simulink model "Udan_SOC"  (R2017b)
settings: Solver=FixedStepAuto  StartTime=0.0  StopTime=1000  FixedStep=0.1  RelTol=1e-3
values from neighbouring files (symbols this model uses):
  DenominatorOfIntegratorFactor = 100.0    [SOC_Stateflow.sldd]
  SOC_CalcSohLKT = 1.0    [SOC_Stateflow.sldd]
  SOC_CalcSOHTempLimit = 70.0    [SOC_Stateflow.sldd]
  SOC_CapPerCycle = 100.0    [SOC_Stateflow.sldd]
  SOC_CapTemp_HLimit = 200.0    [SOC_Stateflow.sldd]
  SOC_CapTemp_LLimit = 0.0    [SOC_Stateflow.sldd]
  Soc_ConfigInfo = 0    [SOC_Stateflow.sldd]
  SOC_DchgEndCalib = 0.0    [SOC_Stateflow.sldd]
  SOC_DiffVoltMin = 10.0    [SOC_Stateflow.sldd]
  SOC_DSOCJumpMax = 500.0    [SOC_Stateflow.sldd]
  SOC_EfficientHighLimit = 250.0    [SOC_Stateflow.sldd]
  SOC_EfficientLowLimit = 40.0    [SOC_Stateflow.sldd]
  SOC_EmptyAus = 0.0    [SOC_Stateflow.sldd]
  SOC_EnableOcv = 1.0    [SOC_Stateflow.sldd]
  SOC_END_CALIB_STATE : value not decoded    [SOC_Stateflow.sldd]
  SOC_HighRealSoc = 95.0    [SOC_Stateflow.sldd]
  SOC_LKTSohCycles = 0.0 1.0 10.0 20.0 30.0 40.0 50.0 60.0 70.0 80.0 90.0 100.0 110.0 120.0 130.0 140.0 150.0 160.0 170.0 180.0 190.0 200.0 210.0 220.0 230.0 240.0 250.0 260.0 270.0 280.0 290.0 300.0 310.0 320.0 330.0 340.0 350.0 360.0 370.0 380.0 390.0 400.0 410.0 420.0 430.0 440.0 450.0 460.0 470.0 480.0 490.0 500.0 510.0 520.0 530.0 540.0 550.0 560.0 570.0 580.0 590.0 600.0 610.0 620.0 630.0 640.0 650.0 660.0 670.0    [SOC_Stateflow.sldd]
  SOC_LKTSohTable = 1000.0 991.0 989.0 992.0 993.0 995.0 994.0 993.0 1000.0 997.0 1002.0 1000.0 992.0 1000.0 989.0 992.0 989.0 994.0 989.0 993.0 994.0 994.0 994.0 993.0 991.0 991.0 992.0 993.0 991.0 985.0 985.0 985.0 979.0 975.0 978.0 984.0 982.0 974.0 975.0 972.0 972.0 975.0 977.0 977.0 974.0 971.0 973.0 971.0 966.0 968.0 965.0 959.0 957.0 956.0 957.0 954.0 955.0 951.0 954.0 951.0 942.0 942.0 940.0 942.0 947.0 949.0    [SOC_Stateflow.sldd]
  SOC_LowRealSoc = 5.0    [SOC_Stateflow.sldd]
  SOC_NominalCap_AmS = 576000000.0    [SOC_Stateflow.sldd]
  SOC_NominalVol = 4000.0    [SOC_Stateflow.sldd]
  SOC_OCVTemp_HLimit = 106.0    [SOC_Stateflow.sldd]
  SOC_OCVTemp_LLimit = 29.0    [SOC_Stateflow.sldd]
  SOC_ShortCalibDSoc = 1.0    [SOC_Stateflow.sldd]
  SOC_SOCResolution = 10000.0    [SOC_Stateflow.sldd]
  SOC_SohCalcCapPercent = 8.0    [SOC_Stateflow.sldd]
  SOC_SohCalcHighLimit = 60.0    [SOC_Stateflow.sldd]
  SOC_SohCalcLowLimit = 10.0    [SOC_Stateflow.sldd]
  SOC_SohCalcMidLimit = 30.0    [SOC_Stateflow.sldd]
  SOC_SOHResolution = 1000.0    [SOC_Stateflow.sldd]
  SOC_State = <binary blob, 1163 chars, not shown>    [SOC_Stateflow.sldd]
  SOC_TempCap_CapBuffer : value not decoded    [SOC_Stateflow.sldd]
  SOC_TempCap_TempBuffer : value not decoded    [SOC_Stateflow.sldd]
  SocOcvCalib_ConfigInfo = 0.0    [SOC_Stateflow.sldd]
  SocOcvCalib_SocBuffer1 : value not decoded    [SOC_Stateflow.sldd]
  SocOcvCalib_TempBuffer : value not decoded    [SOC_Stateflow.sldd]
  SocOcvCalib_VoltageBuffer1 = 3300.0 3303.0 3305.0 3307.0 3310.0 3311.0 3313.0 3314.0 3316.0 3317.0 3319.0 3320.0 3322.0 3323.0 3325.0 3322.0 3323.0 3325.0 3310.0 3313.0 3315.0 3317.0 3320.0 3321.0 3323.0 3324.0 3326.0 3327.0 3329.0 3330.0 3332.0 3333.0 3335.0 3332.0 3333.0 3335.0 3320.0 3323.0 3325.0 3327.0 3330.0 3331.0 3333.0 3334.0 3336.0 3337.0 3339.0 3340.0 3342.0 3343.0 3345.0 3342.0 3343.0 3345.0 3330.0 3333.0 3335.0 3    [SOC_Stateflow.sldd]
  SOHCalibCycle = 10.0    [SOC_Stateflow.sldd]
undefined symbols (not defined in the file or in its folder): DatetimeM_GetReturnType, ParameterM_EeepParaIndexType, Soc_CumuLativeTypeType, SOC_EgthTempChgValue, Soc_EnergyBuffer, SOC_FithTempChgValue, SOC_FstSlowTempChgValue, SOC_FstTempChgValue, SOC_FthTempChgValue, SOC_MaxCap_AmS, SOC_SethTempChgValue, SOC_SixTempChgValue, SOC_SndSlowTempChgValue, SOC_SndTempChgValue, SOC_TrdSlowTempChgValue, SOC_TrdTempChgValue, SocDiagCalib_NoCalibReasonType
libraries: simulink x138, hdlsllib x24, dspindex x4
(part 3 of 10)

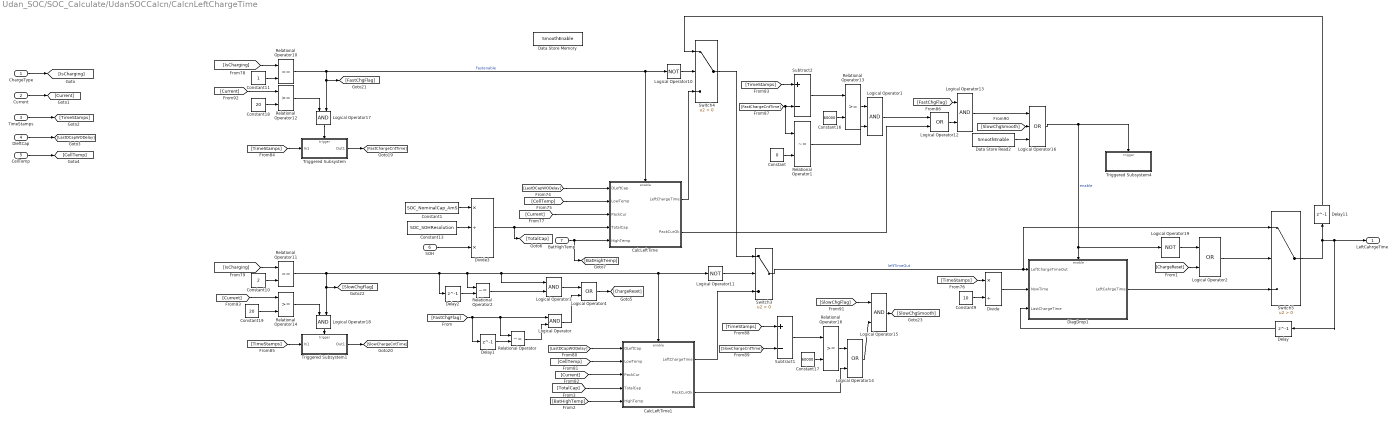
== system Udan_SOC/SOC_Calculate/UdanSOCCalcn/CalcnLeftChargeTime ==
  ChargeType : Inport
  Current : Inport  Port=2
  TimeStamps : Inport  Port=3
  DleftCap : Inport  Port=4
  CellTemp : Inport  Port=5
  SOH : Inport  Port=6
  BatHighTemp : Inport  Port=7
  CalcLeftTime : Subsystem
  CalcLeftTime1 : Subsystem
  Constant : Constant  Value=0  OutDataTypeStr=uint8
  Constant1 : Constant  Value=SOC_NominalCap_AmS
  Constant10 : Constant  Value=2  OutDataTypeStr=uint8
  Constant11 : Constant  OutDataTypeStr=uint8
  Constant13 : Constant  Value=SOC_SOHResolution  OutDataTypeStr=uint16
  Constant16 : Constant  Value=60000  OutDataTypeStr=uint16
  Constant17 : Constant  Value=60000  OutDataTypeStr=uint16
  Constant18 : Constant  Value=20  OutDataTypeStr=uint8
  Constant19 : Constant  Value=20  OutDataTypeStr=uint8
  Constant9 : Constant  Value=10  OutDataTypeStr=uint8
  Data Store Memory : DataStoreMemory  DataStoreName=SmoothEnable  ReadBeforeWriteMsg=warning  WriteAfterWriteMsg=warning  WriteAfterReadMsg=warning  ShowAdditionalParam=off  OutDataTypeStr=boolean
  Data Store Read2 : DataStoreRead  DataStoreName=SmoothEnable
  Delay{,1..2,11} (4 alike) : Delay  DelayLength=1  InitialCondition=0
  DiagDrop1 : Subsystem  mask(DiagDrop(UDAN Lib)){}
      mask help: This block is used to void the slump
  Divide : Product  Inputs=*/  OutDataTypeStr=uint32
  Divide3 : Product  Inputs=*/*  OutDataTypeStr=uint32
  Logical Operator{,1,3,13,15,17..18} (7 alike) : Logic  AllPortsSameDT=off  OutDataTypeStr=boolean
  Logical Operator10 : Logic  Operator=NOT  AllPortsSameDT=off  OutDataTypeStr=boolean
  Logical Operator11 : Logic  Operator=NOT  AllPortsSameDT=off  OutDataTypeStr=boolean
  Logical Operator{2,4,12,14} (4 alike) : Logic  Operator=OR  AllPortsSameDT=off  OutDataTypeStr=boolean
  Logical Operator16 : Logic  Operator=OR  Inputs=3  AllPortsSameDT=off  OutDataTypeStr=boolean
  Logical Operator19 : Logic  Operator=NOT  AllPortsSameDT=off  OutDataTypeStr=boolean
  Relational Operator : RelationalOperator  Operator=~=  OutDataTypeStr=boolean  RndMeth=Simplest
  Relational Operator1 : RelationalOperator  Operator=~=  OutDataTypeStr=boolean  RndMeth=Simplest
  Relational Operator10 : RelationalOperator  Operator===  OutDataTypeStr=boolean  RndMeth=Simplest
  Relational Operator11 : RelationalOperator  Operator===  OutDataTypeStr=boolean  RndMeth=Simplest
  Relational Operator{12..14,16} (4 alike) : RelationalOperator  OutDataTypeStr=boolean  RndMeth=Simplest
  Relational Operator2 : RelationalOperator  Operator=~=  OutDataTypeStr=boolean  RndMeth=Simplest
  Subtract1 : Sum  Inputs=+-  AccumDataTypeStr=uint32  OutDataTypeStr=uint32
  Subtract2 : Sum  Inputs=+-  AccumDataTypeStr=uint32  OutDataTypeStr=uint32
  Switch3 : Switch  Criteria=u2 > Threshold
  Switch4 : Switch  Criteria=u2 > Threshold
  Switch5 : Switch  Criteria=u2 > Threshold
  Triggered Subsystem : Subsystem  TreatAsAtomicUnit=on
  Triggered Subsystem1 : Subsystem  TreatAsAtomicUnit=on
  Triggered Subsystem4 : Subsystem  TreatAsAtomicUnit=on
  LeftCahrgeTime : Outport
  wires:
  Logical Operator2/1 -> Switch5/2
  Logical Operator/1 -> Logical Operator4/2
  Delay1/1 -> Relational Operator/2
  Relational Operator/1 -> Logical Operator/2
  [FastChgFlag] -> Logical Operator/1, Relational Operator/1, Delay1/1
  Delay/1 -> DiagDrop1/3(LastChargeTime)
  Delay11/1 -> Switch4/1
  Switch4/1 -> Switch3/1
  CalcLeftTime/2(PackCurOk) -> Logical Operator12/2
  [Current] -> CalcLeftTime/3(PackCur)
  Relational Operator10/1 -> Logical Operator17/2, [FastChgFlag], Logical Operator10/1, CalcLeftTime/Enable  "Fastenable"
  Constant9/1 -> Divide/2
  [IsCharging] -> Relational Operator10/1
  Constant11/1 -> Relational Operator10/2
  Constant10/1 -> Relational Operator11/2
  Subtract2/1 -> Relational Operator13/1
  Switch5/1 -> Delay11/1, LeftCahrgeTime/1, Delay/1
  [FastChargeCntTime] -> Relational Operator1/1, Subtract2/2
  Relational Operator13/1 -> Logical Operator1/1
  Logical Operator10/1 -> Switch4/2
  [IsCharging] -> Relational Operator11/1
  [Current] -> CalcLeftTime1/3(PackCur)
  [LastDCapWODelay] -> CalcLeftTime1/1(DLeftCap)
  [LastDCapWODelay] -> CalcLeftTime/1(DLeftCap)
  [TimeStamps] -> Triggered Subsystem1/1(In1)
  Triggered Subsystem1/1(Out1) -> [SlowChargeCntTime]
  Triggered Subsystem/1(Out1) -> [FastChargeCntTime]
  [TimeStamps] -> Subtract2/1
  [CellTemp] -> CalcLeftTime1/2(LowTemp)
  Constant16/1 -> Relational Operator13/2
  [CellTemp] -> CalcLeftTime/2(LowTemp)
  Logical Operator15/1 -> [SlowChgSmooth]
  DiagDrop1/1(LeftCahrgeTime) -> Switch5/3
  Switch3/1 -> Switch5/1, DiagDrop1/1(LeftChargeTimeOut)  "leftTimeOut"
  Logical Operator18/1 -> Triggered Subsystem1/Trigger
  Logical Operator13/1 -> Logical Operator16/1
  Logical Operator17/1 -> Triggered Subsystem/Trigger
  [TimeStamps] -> Divide/1
  Relational Operator12/1 -> Logical Operator17/1
  [Current] -> Relational Operator14/1
  [Current] -> Relational Operator12/1
  Constant18/1 -> Relational Operator12/2
  [SlowChgSmooth] -> Logical Operator16/2
  Relational Operator14/1 -> Logical Operator18/1
  Logical Operator19/1 -> Logical Operator2/1
  Logical Operator16/1 -> Triggered Subsystem4/Trigger, Logical Operator19/1, DiagDrop1/Enable  "enable"
  Constant19/1 -> Relational Operator14/2
  [TimeStamps] -> Triggered Subsystem/1(In1)
  Divide/1 -> DiagDrop1/2(NowTime)
  [SlowChargeCntTime] -> Subtract1/2
  CalcLeftTime1/2(PackCurOk) -> Logical Operator14/2
  CalcLeftTime/1(LeftChargeTime) -> Switch4/3
  Logical Operator14/1 -> Logical Operator15/2
  [TimeStamps] -> Subtract1/1
  Relational Operator16/1 -> Logical Operator14/1
  [SlowChgFlag] -> Logical Operator15/1
  Subtract1/1 -> Relational Operator16/1
  Constant17/1 -> Relational Operator16/2
  CalcLeftTime1/1(LeftChargeTime) -> Switch3/3
  Logical Operator12/1 -> Logical Operator13/2
  Logical Operator11/1 -> Switch3/2
  [FastChgFlag] -> Logical Operator13/1
  ChargeType/1 -> [IsCharging]
  Current/1 -> [Current]
  TimeStamps/1 -> [TimeStamps]
  DleftCap/1 -> [LastDCapWODelay]
  CellTemp/1 -> [CellTemp]
  Constant/1 -> Relational Operator1/2
  Relational Operator1/1 -> Logical Operator1/2
  Logical Operator1/1 -> Logical Operator12/1
  Data Store Read2/1 -> Logical Operator16/3
  Relational Operator11/1 -> Delay2/1, Relational Operator2/1, Logical Operator3/1, CalcLeftTime1/Enable, Logical Operator11/1, [SlowChgFlag], Logical Operator18/2
  Delay2/1 -> Relational Operator2/2
  Relational Operator2/1 -> Logical Operator3/2
  Logical Operator3/1 -> Logical Operator4/1
  Logical Operator4/1 -> [ChargeReset]
  [ChargeReset] -> Logical Operator2/2
  SOH/1 -> Divide3/3
  [TotalCap] -> CalcLeftTime1/4(TotalCap)
  Constant13/1 -> Divide3/2
  Constant1/1 -> Divide3/1
  Divide3/1 -> [TotalCap], CalcLeftTime/4(TotalCap)
  BatHighTemp/1 -> [BatHighTemp], CalcLeftTime/5(HighTemp)
  [BatHighTemp] -> CalcLeftTime1/5(HighTemp)

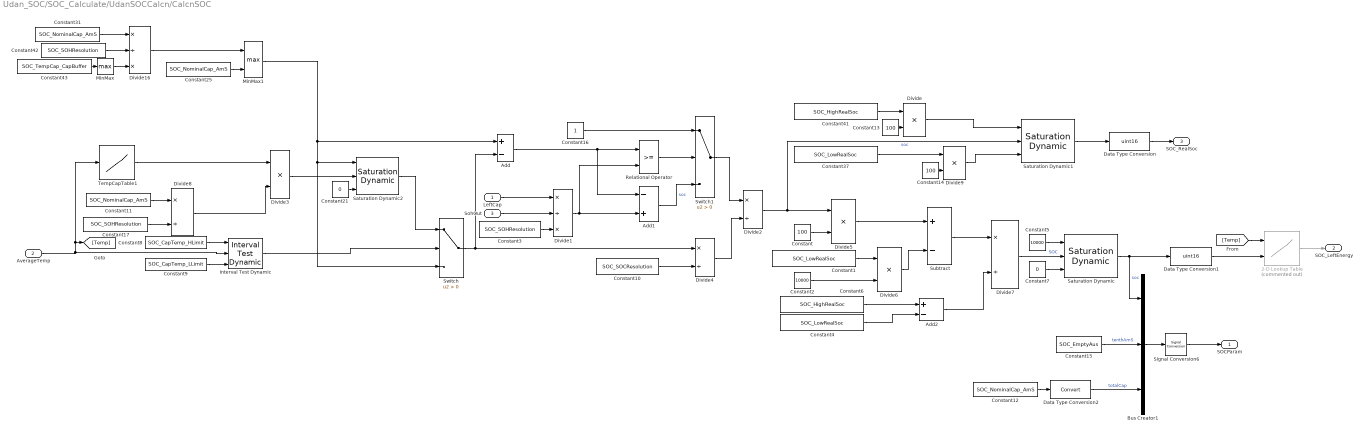
== system Udan_SOC/SOC_Calculate/UdanSOCCalcn/CalcnSOC ==
  LeftCap : Inport
  AverageTemp : Inport  Port=2
  SohOut : Inport  Port=3
  2-D Lookup Table : Lookup_n-D  Commented=on  BreakpointsForDimension1=SocOcvCalib_TempBuffer  BreakpointsForDimension2=SocOcvCalib_SocBuffer1  Table=Soc_EnergyBuffer  ExtrapMethod=Clip  InternalRulePriority=Speed  OutDataTypeStr=uint16  RndMeth=Simplest
  Add : Sum  Inputs=+-
  Add1 : Sum  Inputs=-+  AccumDataTypeStr=uint32  OutDataTypeStr=uint32
  Add2 : Sum  Inputs=+-  AccumDataTypeStr=uint8  OutDataTypeStr=uint8
  Bus Creator1 : BusCreator  Inputs=3  OutDataTypeStr=Bus: SOX_SocType
      settings: InheritFromInputs=off
  Constant : Constant  Value=100  OutDataTypeStr=uint8
  Constant1 : Constant  Value=SOC_LowRealSoc
  Constant10 : Constant  Value=SOC_SOCResolution  OutDataTypeStr=uint16
  Constant{11..12,25,31} (4 alike) : Constant  Value=SOC_NominalCap_AmS
  Constant13 : Constant  Value=100  OutDataTypeStr=uint8
  Constant14 : Constant  Value=100  OutDataTypeStr=uint8
  Constant15 : Constant  Value=SOC_EmptyAus
  Constant16 : Constant  OutDataTypeStr=uint32
  Constant17 : Constant  Value=SOC_SOHResolution  OutDataTypeStr=uint16
  Constant2 : Constant  Value=10000  OutDataTypeStr=uint16
  Constant21 : Constant  Value=0  OutDataTypeStr=uint8
  Constant3 : Constant  Value=SOC_SOHResolution  OutDataTypeStr=uint16
  Constant37 : Constant  Value=SOC_LowRealSoc
  Constant4 : Constant  Value=SOC_LowRealSoc
  Constant41 : Constant  Value=SOC_HighRealSoc
  Constant42 : Constant  Value=SOC_SOHResolution  OutDataTypeStr=uint16
  Constant43 : Constant  Value=SOC_TempCap_CapBuffer
  Constant5 : Constant  Value=10000  OutDataTypeStr=uint16
  Constant6 : Constant  Value=SOC_HighRealSoc
  Constant7 : Constant  Value=0  OutDataTypeStr=uint16
  Constant8 : Constant  Value=SOC_CapTemp_HLimit  OutDataTypeStr=uint8
  Constant9 : Constant  Value=SOC_CapTemp_LLimit  OutDataTypeStr=uint8
  Data Type Conversion : DataTypeConversion  OutDataTypeStr=uint16
  Data Type Conversion1 : DataTypeConversion  OutDataTypeStr=uint16
  Data Type Conversion2 : DataTypeConversion
  Divide : Product  Inputs=**
  Divide1 : Product  Inputs=*/*  OutDataTypeStr=uint32
  Divide16 : Product  Inputs=*/*  OutDataTypeStr=uint32
  Divide2 : Product  Inputs=*/  OutDataTypeStr=int32
  Divide3 : Product  Inputs=**  OutDataTypeStr=uint32
  Divide4 : Product  Inputs=*/  OutDataTypeStr=int32
  Divide5 : Product  Inputs=**  OutDataTypeStr=uint32
  Divide6 : Product  Inputs=**  OutDataTypeStr=uint32
  Divide7 : Product  Inputs=*/  OutDataTypeStr=int32
  Divide8 : Product  Inputs=*/  OutDataTypeStr=uint32
  Divide9 : Product  Inputs=**
  Interval Test Dynamic : simulink/Logic and Bit Operations/Interval Test Dynamic  IntervalClosedRight=off  IntervalClosedLeft=off  OutDataTypeStr=boolean
      settings: SourceProductName=Simulink  SourceProductBaseCode=SL
  MinMax : MinMax  Function=max
  MinMax1 : MinMax  Function=max  Inputs=2
  Relational Operator : RelationalOperator  OutDataTypeStr=boolean  RndMeth=Simplest
  Saturation Dynamic : simulink/Discontinuities/Saturation Dynamic  OutMin=[]  OutMax=[]  OutDataTypeStr=uint32  OutputDataTypeScalingMode=uint32  OutDataType=fixdt(1, 16)  OutScaling=2^-10  DoSatur=on
  Saturation Dynamic1 : simulink/Discontinuities/Saturation Dynamic  OutMin=[]  OutMax=[]  OutDataTypeStr=uint32  OutputDataTypeScalingMode=uint32  OutDataType=fixdt(1, 16)  OutScaling=2^-10  DoSatur=on
  Saturation Dynamic2 : simulink/Discontinuities/Saturation Dynamic  OutMin=[]  OutMax=[]  OutDataTypeStr=Inherit: Same as second input  OutDataType=fixdt(1, 16)  OutScaling=2^-10  DoSatur=off
  Signal Conversion6 : SignalConversion  ConversionOutput=Nonvirtual bus  OverrideOpt=off
  Subtract : Sum  Inputs=+-  AccumDataTypeStr=int32  OutDataTypeStr=int32
  Switch : Switch  Criteria=u2 > Threshold
  Switch1 : Switch  Criteria=u2 > Threshold  OutDataTypeStr=uint32
  TempCapTable1 : Lookup_n-D  NumberOfTableDimensions=1  BreakpointsForDimension1=SOC_TempCap_TempBuffer  Table=SOC_TempCap_CapBuffer  ExtrapMethod=Clip  InternalRulePriority=Speed  OutDataTypeStr=uint16  RndMeth=Simplest  InputSameDT=on
  SOCParam : Outport
  SOC_LeftEnergy : Outport  Port=2
  SOC_RealSoc : Outport  Port=3
  wires:
  Constant15/1 -> Bus Creator1/2  "tenthAmS"
  LeftCap/1 -> Divide1/1
  Constant10/1 -> Divide4/2
  TempCapTable1/1 -> Divide3/1
  Constant3/1 -> Divide1/3
  Divide7/1 -> Saturation Dynamic/2  "SOC"
  Constant7/1 -> Saturation Dynamic/3
  Constant5/1 -> Saturation Dynamic/1
  SohOut/1 -> Divide1/2
  Saturation Dynamic/1 -> Data Type Conversion1/1, Bus Creator1/1  "soc"
  Divide4/1 -> Divide2/2
  Signal Conversion6/1 -> SOCParam/1
  Bus Creator1/1 -> Signal Conversion6/1
  Switch/1 -> Add/2, Divide4/1
  Divide8/1 -> Divide3/2
  AverageTemp/1 -> [Temp], TempCapTable1/1, Interval Test Dynamic/2
  Constant9/1 -> Interval Test Dynamic/3
  Constant8/1 -> Interval Test Dynamic/1
  Interval Test Dynamic/1 -> Switch/2
  Saturation Dynamic2/1 -> Switch/1
  MinMax1/1 -> Add/1, Saturation Dynamic2/1, Switch/3
  Divide1/1 -> Relational Operator/2, Add1/2
  Add/1 -> Add1/1, Relational Operator/1
  Constant17/1 -> Divide8/2
  Divide2/1 -> Divide5/1, Saturation Dynamic1/2  "soc"
  Data Type Conversion1/1 -> 2-D Lookup Table/2
  [Temp] -> 2-D Lookup Table/1
  2-D Lookup Table/1 -> SOC_LeftEnergy/1
  Data Type Conversion/1 -> SOC_RealSoc/1
  Saturation Dynamic1/1 -> Data Type Conversion/1
  Divide3/1 -> Saturation Dynamic2/2
  Constant21/1 -> Saturation Dynamic2/3
  Constant/1 -> Divide5/2
  Divide5/1 -> Subtract/1
  Constant2/1 -> Divide6/2
  Divide6/1 -> Subtract/2
  Subtract/1 -> Divide7/1
  Add2/1 -> Divide7/2
  Constant13/1 -> Divide/2
  Divide/1 -> Saturation Dynamic1/1
  Constant14/1 -> Divide9/2
  Divide9/1 -> Saturation Dynamic1/3
  Data Type Conversion2/1 -> Bus Creator1/3  "totalCap"
  Constant11/1 -> Divide8/1
  Constant12/1 -> Data Type Conversion2/1
  Constant41/1 -> Divide/1
  Constant37/1 -> Divide9/1
  Constant1/1 -> Divide6/1
  Constant6/1 -> Add2/1
  Constant4/1 -> Add2/2
  Relational Operator/1 -> Switch1/2
  Constant16/1 -> Switch1/1
  Add1/1 -> Switch1/3  "soc"
  Switch1/1 -> Divide2/1
  Constant42/1 -> Divide16/2
  Constant43/1 -> MinMax/1
  MinMax/1 -> Divide16/3
  Divide16/1 -> MinMax1/1
  Constant25/1 -> MinMax1/2
  Constant31/1 -> Divide16/1

== system Udan_SOC/SOC_Calculate/UdanSOCCalcn/CalcnSOC1 ==
  LeftCap : Inport
  Current : Inport  Port=2
  FullCharge : Inport  Port=3
  AverageTemp : Inport  Port=4
  SohOut : Inport  Port=5
  TempCapResolution : Inport  Port=6
  IsCharging : Inport  Port=7
  Abs : Abs
  Add : Sum  Inputs=+-
  Add1 : Sum  Inputs=-+  AccumDataTypeStr=uint32  OutDataTypeStr=uint32
  Bus Creator1 : BusCreator  Inputs=3  OutDataTypeStr=Bus: SOX_SocType
      settings: InheritFromInputs=off
  Constant1 : Constant  Commented=on  Value=10000  OutDataTypeStr=uint16
  Constant10 : Constant  Value=SOC_SOCResolution  OutDataTypeStr=uint16
  Constant{4,6,11,16} (4 alike) : Constant  Value=SOC_NominalCap_AmS
  Constant12 : Constant  Commented=on  Value=9900  OutDataTypeStr=uint16
  Constant13 : Constant  Commented=on  Value=9900  OutDataTypeStr=uint16
  Constant14 : Constant  Value=0  OutDataTypeStr=uint32
  Constant15 : Constant  Value=SOC_EmptyAus
  Constant17 : Constant  Value=SOC_SOHResolution  OutDataTypeStr=uint16
  Constant18 : Constant  Value=SOC_SOHResolution  OutDataTypeStr=uint16
  Constant2 : Constant  Commented=on  Value=2  OutDataTypeStr=int8
  Constant3 : Constant  Value=SOC_SOHResolution  OutDataTypeStr=uint16
  Constant5 : Constant  Value=10000  OutDataTypeStr=uint16
  Constant7 : Constant  Value=0  OutDataTypeStr=uint16
  Constant8 : Constant  Value=SOC_CapTemp_HLimit  OutDataTypeStr=uint8
  Constant9 : Constant  Value=SOC_CapTemp_LLimit  OutDataTypeStr=uint8
  Data Type Conversion : DataTypeConversion
  Delay10 : Delay  Commented=on  DelayLength=1  InitialCondition=0
  Divide1 : Product  Inputs=*/*  OutDataTypeStr=uint32
  Divide2 : Product  Inputs=*/  OutDataTypeStr=int32
  Divide3 : Product  Inputs=**  OutDataTypeStr=uint32
  Divide4 : Product  Inputs=*/  OutDataTypeStr=int32
  Divide8 : Product  Inputs=*/  OutDataTypeStr=uint32
  Interval Test Dynamic : simulink/Logic and Bit Operations/Interval Test Dynamic  IntervalClosedRight=off  IntervalClosedLeft=off  OutDataTypeStr=boolean
      settings: SourceProductName=Simulink  SourceProductBaseCode=SL
  Logical Operator : Logic  Commented=on  Operator=NOT  AllPortsSameDT=off  OutDataTypeStr=boolean
  Logical Operator1 : Logic  Commented=on  AllPortsSameDT=off  OutDataTypeStr=boolean
  Logical Operator2 : Logic  Commented=on  AllPortsSameDT=off  OutDataTypeStr=boolean
  Logical Operator3 : Logic  Commented=on  AllPortsSameDT=off  OutDataTypeStr=boolean
  Logical Operator4 : Logic  Commented=on  Operator=NOT  AllPortsSameDT=off  OutDataTypeStr=boolean
  Relational Operator : RelationalOperator  Commented=on  OutDataTypeStr=boolean  RndMeth=Simplest
  Relational Operator1 : RelationalOperator  Commented=on  OutDataTypeStr=boolean  RndMeth=Simplest
  Saturation Dynamic : simulink/Discontinuities/Saturation Dynamic  OutMin=[]  OutMax=[]  OutDataTypeStr=uint32  OutputDataTypeScalingMode=uint32  OutDataType=fixdt(1, 16)  OutScaling=2^-10  DoSatur=on
  Signal Conversion6 : SignalConversion  ConversionOutput=Nonvirtual bus  OverrideOpt=off
  Switch : Switch  Criteria=u2 > Threshold
  Switch1 : Switch  Commented=on  Criteria=u2 > Threshold  OutDataTypeStr=int16
  Switch3 : Switch  Criteria=u2 > Threshold  OutDataTypeStr=int32
  Switch6 : Switch  Commented=on  Criteria=u2 > Threshold  OutDataTypeStr=int16
  TempCapTable1 : Lookup_n-D  Commented=on  NumberOfTableDimensions=1  BreakpointsForDimension1=SOC_TempCap_TempBuffer  Table=SOC_TempCap_CapBuffer  ExtrapMethod=Clip  InternalRulePriority=Speed  OutDataTypeStr=uint16  RndMeth=Simplest  InputSameDT=on
  Terminator : Terminator
  SOCParam : Outport
  wires:
  TempCapResolution/1 -> Terminator/1
  Constant15/1 -> Bus Creator1/2  "tenthAmS"
  Data Type Conversion/1 -> Bus Creator1/3  "totalCap"
  LeftCap/1 -> Divide1/1
  Constant10/1 -> Divide4/2
  TempCapTable1/1 -> ?
  Constant3/1 -> Divide1/3
  Switch1/1 -> ?  "SOC"
  Constant7/1 -> Saturation Dynamic/3
  Constant5/1 -> Saturation Dynamic/1
  SohOut/1 -> Divide1/2
  Constant1/1 -> Switch1/1
  Switch6/1 -> Switch1/3
  Saturation Dynamic/1 -> Bus Creator1/1  "soc"
  Divide4/1 -> Divide2/2
  Signal Conversion6/1 -> SOCParam/1
  Add1/1 -> Divide2/1  "soc"
  Bus Creator1/1 -> Signal Conversion6/1
  Switch/1 -> Add/1, Divide4/1
  AverageTemp/1 -> TempCapTable1/1, Interval Test Dynamic/2
  Constant9/1 -> Interval Test Dynamic/3
  Constant8/1 -> Interval Test Dynamic/1
  Interval Test Dynamic/1 -> Switch/2
  Divide3/1 -> Switch/1
  Constant11/1 -> Switch/3
  Constant4/1 -> Add/2
  Constant14/1 -> Switch3/1
  Add/1 -> Switch3/2, Switch3/3
  Divide1/1 -> Add1/2
  Switch3/1 -> Abs/1
  Abs/1 -> Add1/1
  Constant16/1 -> Divide8/1
  Constant17/1 -> Divide8/2
  Divide8/1 -> Divide3/2
  Constant18/1 -> Divide3/1
  Logical Operator2/1 -> Switch1/2
  Constant2/1 -> Relational Operator/2
  Relational Operator/1 -> Logical Operator1/2
  ? -> Relational Operator1/1, Switch6/1  "soc"
  Constant13/1 -> Relational Operator1/2
  Relational Operator1/1 -> Logical Operator1/1
  IsCharging/1 -> Logical Operator2/2
  Current/1 -> Relational Operator/1
  Logical Operator1/1 -> Logical Operator/1
  Constant12/1 -> Switch6/3
  Logical Operator/1 -> Switch6/2
  FullCharge/1 -> Delay10/1, Logical Operator3/1
  Delay10/1 -> Logical Operator4/1
  Logical Operator4/1 -> Logical Operator3/2
  Logical Operator3/1 -> Logical Operator2/1
  Divide2/1 -> Saturation Dynamic/2  "soc"
  Constant6/1 -> Data Type Conversion/1  "totalCap"

== system Udan_SOC/SOC_Calculate/UdanSOCCalcn/CalibEmptySOC ==
  Capacity : Inport
  SOH : Inport  Port=2
  AverageTemp : Inport  Port=3
  EmptyValue : Inport  Port=4
  function : TriggerPort  TriggerType=function-call  VariantControl=Variant
  Constant : Constant  Value=10  OutDataTypeStr=uint8
  Constant1 : Constant  Value=SOC_NominalCap_AmS
  Constant2 : Constant  Value=SOC_SOCResolution
  Constant3 : Constant  Value=2  OutDataTypeStr=uint8
  Constant31 : Constant  Value=SOC_NominalCap_AmS
  Constant37 : Constant  Value=SOC_LowRealSoc
  Constant5 : Constant  Value=100  OutDataTypeStr=uint8
  ConvertSOC2AH : Subsystem
  Divide : Product  Inputs=**  OutDataTypeStr=uint32
  Divide1 : Product  Inputs=*/*  OutDataTypeStr=uint32
  Divide2 : Product  Inputs=**  OutDataTypeStr=uint16
  Divide3 : Product  Inputs=**
  MinMax : MinMax  Function=max  Inputs=2  OutDataTypeStr=uint32
  MinMax1 : MinMax  Function=max  Inputs=2
  MinMax2 : MinMax  Function=max  Inputs=2
  Terminator : Terminator
  NewCap : Outport
  NewDCap : Outport  Port=2
  wires:
  MinMax/1 -> Terminator/1  "AmS"
  SOH/1 -> [SOH], Divide/2
  Divide/1 -> MinMax/2
  Capacity/1 -> MinMax/1
  Divide1/1 -> NewDCap/1  "AmS"
  Constant31/1 -> Divide1/1
  Constant2/1 -> Divide1/2
  Constant/1 -> Divide2/2
  ConvertSOC2AH/1(AHOut) -> NewCap/1  "AmS"
  AverageTemp/1 -> [TCell]
  MinMax2/1 -> ConvertSOC2AH/2(SOC)
  [SOH] -> ConvertSOC2AH/3(SOH)
  [TCell] -> ConvertSOC2AH/1(BatTemp)
  Constant5/1 -> Divide3/2
  Constant1/1 -> Divide/1
  Constant37/1 -> Divide3/1
  EmptyValue/1 -> Divide2/1
  MinMax1/1 -> Divide1/3
  Divide2/1 -> MinMax1/1, MinMax2/1
  Constant3/1 -> MinMax1/2
  Divide3/1 -> MinMax2/2

== system Udan_SOC/SOC_Calculate/UdanSOCCalcn/CalibFullSOC ==
  Capacity : Inport
  SOH : Inport  Port=2
  BatTemp : Inport  Port=3
  function : TriggerPort  TriggerType=function-call  VariantControl=Variant
  Add : Sum  Inputs=+-
  Constant : Constant  Value=0  OutDataTypeStr=uint8
  Constant1 : Constant  Commented=on  Value=0  OutDataTypeStr=uint32
  Constant19 : Constant  Value=SOC_SOCResolution  OutDataTypeStr=uint16
  Constant{2,4,24,42} (4 alike) : Constant  Value=SOC_SOHResolution  OutDataTypeStr=uint16
  Constant{3,5,25,31} (4 alike) : Constant  Value=SOC_NominalCap_AmS
  Constant41 : Constant  Value=SOC_HighRealSoc
  Constant43 : Constant  Value=SOC_TempCap_CapBuffer
  Constant9 : Constant  Value=100  OutDataTypeStr=uint8
  DchgPower2 : simulink/Sources/Enumerated Constant  Commented=on  OutDataTypeStr=Enum: ParameterM_EeepParaIndexType  Value=ParameterM_EeepParaIndexType.PARAMETERM_EEEP_LEFTCAP_WOCALIB_H_INDEX  SampleTime=inf
      settings: SourceProductName=Simulink
  DchgPower4 : simulink/Sources/Enumerated Constant  Commented=on  OutDataTypeStr=Enum: ParameterM_EeepParaIndexType  Value=ParameterM_EeepParaIndexType.PARAMETERM_EEEP_LEFTCAP_WOCALIB_L_INDEX  SampleTime=inf
      settings: SourceProductName=Simulink
  Divide : Product  Inputs=**  OutDataTypeStr=uint32
  Divide1 : Product  Inputs=*/  OutDataTypeStr=uint32
  Divide16 : Product  Inputs=*/*  OutDataTypeStr=uint32
  Divide2 : Product  Inputs=**  OutDataTypeStr=uint32
  Divide3 : Product  Inputs=*/  OutDataTypeStr=uint32
  Divide4 : Product  Inputs=*/*  OutDataTypeStr=int32  RndMeth=Round
  Divide5 : Product  Inputs=**  OutDataTypeStr=uint32
  Divide7 : Product  Inputs=**
  Divide8 : Product  Inputs=*/  OutDataTypeStr=uint32
  MinMax : MinMax  Function=max  OutDataTypeStr=uint32
  MinMax1 : MinMax  Function=max
  MinMax2 : MinMax  Function=max  Inputs=2
  Saturation Dynamic : simulink/Discontinuities/Saturation Dynamic  OutMin=[]  OutMax=[]  OutDataTypeStr=Inherit: Same as second input  OutDataType=fixdt(1, 16)  OutScaling=2^-10  DoSatur=off
  Subsystem : Subsystem  Commented=on  mask(EeepWrite_uint32){}
      mask help: EeepWrite_uint32
  Subtract : Sum  Inputs=+-  AccumDataTypeStr=int32  OutDataTypeStr=int32
  TempCapTable1 : Lookup_n-D  NumberOfTableDimensions=1  BreakpointsForDimension1=SOC_TempCap_TempBuffer  Table=SOC_TempCap_CapBuffer  ExtrapMethod=Clip  InternalRulePriority=Speed  OutDataTypeStr=uint16  RndMeth=Simplest  InputSameDT=on
  Terminator : Terminator
  NewCap : Outport
  NewDCap : Outport  Port=2
  wires:
  Constant2/1 -> Divide1/2
  Divide1/1 -> Divide/1
  SOH/1 -> [SOH], Divide2/2
  Constant3/1 -> Divide1/1
  Divide/1 -> MinMax/1
  Capacity/1 -> Terminator/1
  MinMax/1 -> NewDCap/1  "AmS"
  DchgPower4/1 -> Subsystem/3(LowIndex)
  DchgPower2/1 -> Subsystem/2(HighIndex)
  Constant1/1 -> Subsystem/1(data)
  Constant4/1 -> Divide3/2
  Divide3/1 -> Divide2/1
  [SOH] -> Divide/2
  Constant19/1 -> Add/1, Divide4/2  "SOC"
  BatTemp/1 -> TempCapTable1/1
  TempCapTable1/1 -> Divide5/1
  Divide8/1 -> Divide5/2
  Constant5/1 -> Divide8/1
  Constant24/1 -> Divide8/2
  Saturation Dynamic/1 -> Divide4/1
  Divide4/1 -> Subtract/2
  MinMax2/1 -> Subtract/1, Saturation Dynamic/1  "soc"
  Divide2/1 -> NewCap/1
  Divide5/1 -> Saturation Dynamic/2
  Constant/1 -> Saturation Dynamic/3
  Add/1 -> Divide4/3
  Divide7/1 -> Add/2
  Constant9/1 -> Divide7/2
  Constant41/1 -> Divide7/1
  Subtract/1 -> Divide3/1
  Constant42/1 -> Divide16/2
  Constant43/1 -> MinMax1/1
  MinMax1/1 -> Divide16/3
  Divide16/1 -> MinMax2/1
  Constant25/1 -> MinMax2/2
  Constant31/1 -> Divide16/1

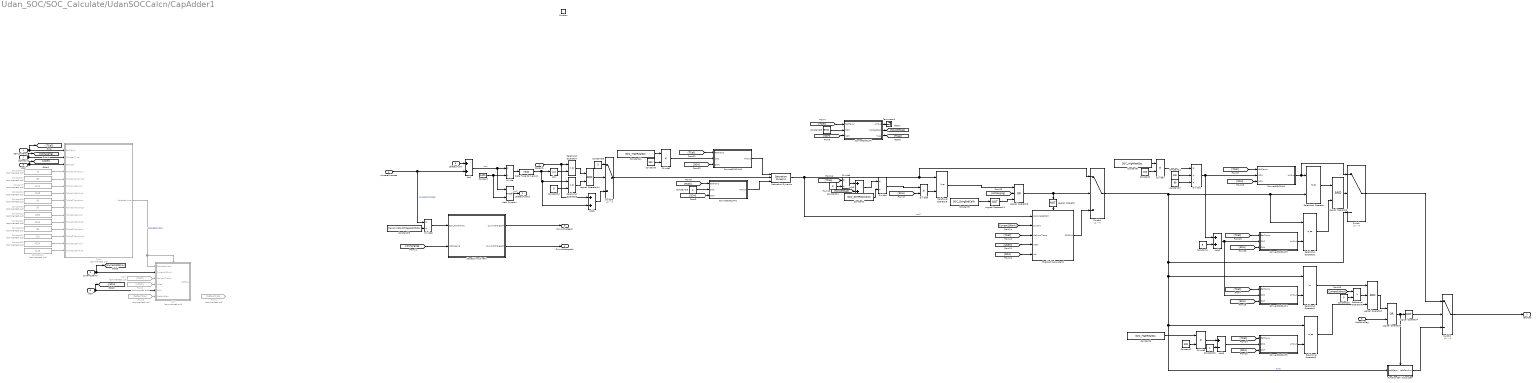
== system Udan_SOC/SOC_Calculate/UdanSOCCalcn/CapAdder1 ==
  Capacity : Inport
  AmpereMicrosec : Inport  Port=2
  Current100mA : Inport  Port=3
  CellLowTemp : Inport  Port=4
  UCell : Inport  Port=5
  SOH : Inport  Port=6
  IsCharging : Inport  Port=7
  LeftCapAusIn : Inport  Port=8
  SocCalibFlag : Inport  Port=9  OutDataTypeStr=uint8  PortDimensions=[1]
  function : TriggerPort  TriggerType=function-call  VariantControl=Variant
  Abs : Abs
  Add : Sum  AccumDataTypeStr=int32  OutDataTypeStr=int32
  Add2 : Sum
  Add3 : Sum  AccumDataTypeStr=uint32  OutDataTypeStr=uint32
  Add5 : Sum  Inputs=+-
  Add6 : Sum  AccumDataTypeStr=uint32  OutDataTypeStr=uint32
  Chart : Stateflow chart  Commented=on  TreatAsAtomicUnit=on
  Constant : Constant  Value=1000  OutDataTypeStr=int32
  Constant1 : Constant  Value=SOC_SOHResolution  OutDataTypeStr=uint16
  Constant10 : Constant  Commented=on  Value=4138  OutDataTypeStr=uint16
  Constant{2..3,5,11} (4 alike) : Constant  Value=100  OutDataTypeStr=uint8
  Constant12 : Constant  Commented=on  Value=4135  OutDataTypeStr=uint16
  Constant13 : Constant  Commented=on  Value=4053  OutDataTypeStr=uint16
  Constant14 : Constant  Commented=on  Value=4118  OutDataTypeStr=uint16
  Constant15 : Constant  Commented=on  Value=4024  OutDataTypeStr=uint16
  Constant16 : Constant  Commented=on  Value=70  OutDataTypeStr=uint8
  Constant17 : Constant  Commented=on  Value=90  OutDataTypeStr=uint8
  Constant18 : Constant  Commented=on  Value=90  OutDataTypeStr=uint8
  Constant19 : Constant  Commented=on  Value=95  OutDataTypeStr=uint8
  Constant20 : Constant  Commented=on  Value=95  OutDataTypeStr=uint8
  Constant21 : Constant  Commented=on  Value=102  OutDataTypeStr=uint8
  Constant22 : Constant  OutDataTypeStr=uint8
  Constant23 : Constant  Value=2  OutDataTypeStr=uint16
  Constant24 : Constant  Value=3  OutDataTypeStr=uint8
  Constant25 : Constant  Value=9702  OutDataTypeStr=uint16
  Constant27 : Constant  Value=99  OutDataTypeStr=uint8
  Constant28 : Constant  Value=0  OutDataTypeStr=uint8
  Constant29 : Constant  Value=DenominatorOfIntegratorFactor  OutDataTypeStr=uint16
  Constant34 : Constant  Value=0  OutDataTypeStr=uint8
  Constant35 : Constant  Value=0  OutDataTypeStr=uint8
  Constant4 : Constant  Value=8  OutDataTypeStr=uint8
  Constant41 : Constant  Value=SOC_HighRealSoc
  Constant6 : Constant  Value=SOC_HighRealSoc
  Constant7 : Constant  Commented=on  Value=4110  OutDataTypeStr=uint16
  Constant8 : Constant  Value=SOC_HighRealSoc
  Constant9 : Constant  Value=SOC_DchgEndCalib
  ConvertSOC2AH : Subsystem
  ConvertSOC2AH1 : Subsystem
  ConvertSOC2AH2 : Subsystem
  ConvertSOC2AH3 : Subsystem
  ConvertSOC2AH4 : Subsystem
  ConvertSOC2AH5 : Subsystem
  ConvertSOC2AH6 : Subsystem
  Data Type Conversion : DataTypeConversion  OutDataTypeStr=int32
  Divide : Product  Inputs=*/  OutDataTypeStr=int32
  Divide1 : Product  Inputs=*/*
  Divide2 : Product  Inputs=**
  Divide3 : Product  Inputs=*/  OutDataTypeStr=uint32
  Divide4 : Product  Inputs=*/  OutDataTypeStr=uint32
  Divide5 : Product  Inputs=**  OutDataTypeStr=uint32
  Divide7 : Product  Inputs=**
  Divide8 : Product  Inputs=**
  Divide9 : Product  Inputs=*/  OutDataTypeStr=int32
  Enabled Subsystem1 : Subsystem  TreatAsAtomicUnit=on
  From : From  Commented=on  GotoTag=TCell
  From1 : From  Commented=on  GotoTag=UCell
  From2 : From  Commented=on  GotoTag=DefaultCap
  From3 : From  Commented=on  GotoTag=DefaultCap
  Function-Call Subsystem : Subsystem  TreatAsAtomicUnit=on
  LKT : Subsystem  Commented=on
  Logical Operator : Logic  Operator=NOT  AllPortsSameDT=off  OutDataTypeStr=boolean
  Logical Operator11 : Logic  Operator=NOT  AllPortsSameDT=off  OutDataTypeStr=boolean
  Logical Operator14 : Logic  AllPortsSameDT=off  OutDataTypeStr=boolean
  Logical Operator3 : Logic  Inputs=3  AllPortsSameDT=off  OutDataTypeStr=boolean
  Logical Operator4 : Logic  Operator=NOT  AllPortsSameDT=off  OutDataTypeStr=boolean
  Logical Operator5 : Logic  Operator=OR  AllPortsSameDT=off  OutDataTypeStr=boolean
  Logical Operator6 : Logic  AllPortsSameDT=off  OutDataTypeStr=boolean
  Logical Operator8 : Logic  Operator=OR  Inputs=3  AllPortsSameDT=off  OutDataTypeStr=boolean
  Math Function : Math  Operator=mod  SaturateOnIntegerOverflow=on
  Relational Operator{,2,5,7..8} (5 alike) : RelationalOperator  Operator=<=  OutDataTypeStr=boolean  RndMeth=Simplest
  Relational Operator1 : RelationalOperator  Operator=>  OutDataTypeStr=boolean  RndMeth=Simplest
  Relational Operator3 : RelationalOperator  OutDataTypeStr=boolean  RndMeth=Simplest
  Relational Operator6 : RelationalOperator  Operator=>  OutDataTypeStr=boolean  RndMeth=Simplest
  Saturation Dynamic : simulink/Discontinuities/Saturation Dynamic  OutMin=[]  OutMax=[]  OutDataTypeStr=uint32  OutputDataTypeScalingMode=uint32  OutDataType=fixdt(1, 16)  OutScaling=2^-10  DoSatur=on
  StoreCulumutiveAh : Subsystem  TreatAsAtomicUnit=on
  Switch : Switch  Criteria=u2 > Threshold
  Switch1 : Switch  Criteria=u2 > Threshold
  Switch4 : Switch  Criteria=u2 > Threshold
  Switch5 : Switch  Criteria=u2 > Threshold  OutDataTypeStr=uint32
  Terminator2 : Terminator
  NewCap : Outport
  LeftCapAusOut : Outport  Port=2
  CulumChargeAh : Outport  Port=3
  CulumDchargeAh : Outport  Port=4
  wires:
  Add/1 -> Divide/1, Math Function/1  "Aus"
  AmpereMicrosec/1 -> Divide9/1, Add/2  "AmpereMicrosec"
  ConvertSOC2AH6/1(AHOut) -> Saturation Dynamic/1
  Divide/1 -> Data Type Conversion/1
  Constant/1 -> Divide/2, Math Function/2
  LeftCapAusIn/1 -> Add/1
  Current100mA/1 -> [Current100mA], LKT/2(Current100mA)
  UCell/1 -> [UCell], Chart/3(BatUCell)
  Saturation Dynamic/1 -> Enabled Subsystem1/1(CalculatedSOC), Switch4/1, Relational Operator3/1  "AmS"
  Math Function/1 -> LeftCapAusOut/1  "AuS"
  IsCharging/1 -> [IsCharging], Chart/2(ChargerType)
  CellLowTemp/1 -> Chart/1(BatTemp), [TCell]
  Chart/1(SelectedIndex) -> LKT/1(SelectedIndex), LKT/Enable  "SelectedIndex"
  Constant7/1 -> Chart/6(Table1UCellLow)
  Constant10/1 -> Chart/7(Table1UCellHigh)
  Constant13/1 -> Chart/10(Table2UCellLow)
  Constant12/1 -> Chart/11(Table2UCellHigh)
  Constant15/1 -> Chart/14(Table3UCellLow)
  Constant14/1 -> Chart/15(Table3UCellHigh)
  Constant16/1 -> Chart/4(Table1TempLow)
  Constant17/1 -> Chart/5(Table1TempHigh)
  Constant18/1 -> Chart/8(Table2TempLow)
  Constant19/1 -> Chart/9(Table2TempHigh)
  Constant20/1 -> Chart/12(Table3TempLow)
  Constant21/1 -> Chart/13(Table3TempHigh)
  SOH/1 -> [SOH], LKT/5(SOH)
  From/1 -> LKT/3(CellLowTemp)
  From1/1 -> LKT/4(UCell)
  From3/1 -> LKT/6(DefaultCap)
  Constant25/1 -> ConvertSOC2AH/2(SOC)
  [TCell] -> ConvertSOC2AH/1(BatTemp)
  [SOH] -> ConvertSOC2AH/3(SOH)
  Constant23/1 -> ConvertSOC2AH2/2(SOC)
  [SOH] -> ConvertSOC2AH2/3(SOH)
  [TCell] -> ConvertSOC2AH2/1(BatTemp)
  [SOH] -> Enabled Subsystem1/5(soh)
  [UCell] -> Enabled Subsystem1/4(UCell)
  [TCell] -> Enabled Subsystem1/3(CellLowTemp)
  [Current100mA] -> Enabled Subsystem1/2(Current)
  Add3/1 -> Divide4/1
  [NoUsedCap] -> Add3/2
  Divide5/1 -> Relational Operator3/2
  Constant24/1 -> Divide3/2
  [TCap] -> Divide3/1
  Divide3/1 -> Add3/1
  Constant1/1 -> Divide4/2
  Divide4/1 -> Divide5/1
  [SOH] -> Divide5/2
  ConvertSOC2AH/3(Tcap) -> [TCap]
  ConvertSOC2AH/2(NoUsedCap) -> [NoUsedCap]
  ConvertSOC2AH/1(AHOut) -> Terminator2/1
  [IsCharging] -> Logical Operator8/2
  Relational Operator3/1 -> Logical Operator8/1
  Logical Operator/1 -> Enabled Subsystem1/Enable
  Logical Operator8/1 -> Switch4/2, Logical Operator/1
  Enabled Subsystem1/1(SOCOut) -> Switch4/3
  Logical Operator3/1 -> Logical Operator5/1
  Logical Operator5/1 -> Logical Operator4/1, Function-Call Subsystem/Trigger
  Switch/1 -> Switch1/1
  Switch1/1 -> NewCap/1
  Add2/1 -> ConvertSOC2AH4/2(SOC), ConvertSOC2AH3/2(SOC)
  ConvertSOC2AH5/1(AHOut) -> Relational Operator5/2
  ConvertSOC2AH3/1(AHOut) -> Relational Operator2/2
  [SOH] -> ConvertSOC2AH3/3(SOH)
  SocCalibFlag/1 -> Logical Operator5/2
  [TCell] -> ConvertSOC2AH3/1(BatTemp)
  [TCell] -> ConvertSOC2AH5/1(BatTemp)
  [TCell] -> ConvertSOC2AH4/1(BatTemp)
  Switch4/1 -> Relational Operator2/1, Relational Operator/2, Switch/3, Relational Operator1/1, Relational Operator5/1, Function-Call Subsystem/1(LeftCapIn)  "AmS"
  Function-Call Subsystem/1(LeftCapOut) -> Switch1/3
  ConvertSOC2AH4/1(AHOut) -> Relational Operator1/2
  [SOH] -> ConvertSOC2AH5/3(SOH)
  ConvertSOC2AH1/1(AHOut) -> Switch/1, Relational Operator/1
  Relational Operator5/1 -> Logical Operator3/3
  Relational Operator6/1 -> Logical Operator3/2
  Logical Operator6/1 -> Switch/2
  [TCell] -> ConvertSOC2AH1/1(BatTemp)
  [SOH] -> ConvertSOC2AH4/3(SOH)
  Relational Operator2/1 -> Logical Operator6/2
  Logical Operator4/1 -> Switch1/2
  Divide1/1 -> ConvertSOC2AH1/2(SOC), Add2/1
  Relational Operator/1 -> Logical Operator6/1
  Relational Operator1/1 -> Logical Operator3/1
  Add5/1 -> ConvertSOC2AH5/2(SOC)
  [SOH] -> ConvertSOC2AH1/3(SOH)
  [SOH] -> ConvertSOC2AH6/3(SOH)
  [TCell] -> ConvertSOC2AH6/1(BatTemp)
  Divide7/1 -> Divide1/1
  Constant11/1 -> Divide1/2
  Constant27/1 -> Divide1/3
  Constant4/1 -> Add2/2
  Constant22/1 -> Add5/2
  Divide8/1 -> Add5/1
  Logical Operator11/1 -> Logical Operator8/3
  Constant3/1 -> Divide2/2
  Divide2/1 -> ConvertSOC2AH6/2(SOC)
  Constant2/1 -> Divide7/2
  Constant5/1 -> Divide8/2
  Constant41/1 -> Divide2/1
  Constant8/1 -> Divide7/1
  Constant6/1 -> Divide8/1
  Constant9/1 -> Logical Operator11/1
  [Current100mA] -> Relational Operator6/1
  Constant28/1 -> Relational Operator6/2
  ConvertSOC2AH2/1(AHOut) -> Saturation Dynamic/3
  Logical Operator14/1 -> Switch5/2
  Relational Operator8/1 -> Logical Operator14/2
  Abs/1 -> Relational Operator7/2
  Add6/1 -> Switch5/3
  Constant35/1 -> Switch5/1
  Capacity/1 -> Add6/1, Relational Operator7/1
  Relational Operator7/1 -> Logical Operator14/1
  Data Type Conversion/1 -> Add6/2, Relational Operator8/1, Abs/1
  Constant34/1 -> Relational Operator8/2
  Switch5/1 -> Saturation Dynamic/2
  Divide9/1 -> StoreCulumutiveAh/1(Cap_TenthAmS)
  [IsCharging] -> StoreCulumutiveAh/2(IsCharging)
  Constant29/1 -> Divide9/2
  StoreCulumutiveAh/1(CulumChargeAh) -> CulumChargeAh/1
  StoreCulumutiveAh/2(CulumDchargeAh) -> CulumDchargeAh/1
